simulink model "MIMO"  (R2024a)
settings: Solver=VariableStepAuto  StartTime=0.0  StopTime=20  RelTol=1e-3
undefined symbols (not defined in the file or in its folder): BOOL, DINT, slplc
(part 1 of 5)
settings Model: PLCLadderLogicAnimation=on  Creator=Jack Vranicar  LastModifiedBy=Jack Vranicar

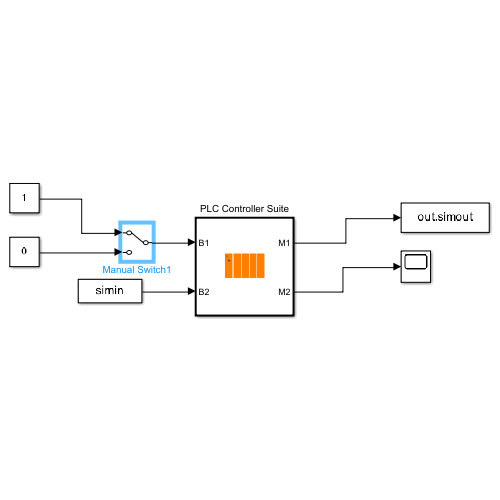
[thumbnail: Simulink's stored preview of the top-level diagram]
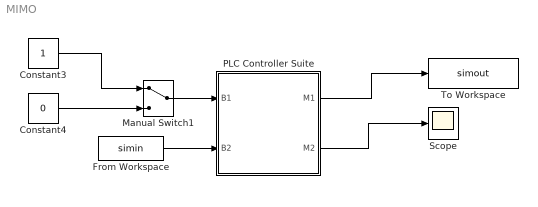
== system MIMO ==
  Constant3 : Constant  OutDataTypeStr=boolean
  Constant4 : Constant  Value=0  OutDataTypeStr=boolean
  From Workspace : FromWorkspace  VariableName=simin
  Manual Switch1 : ManualSwitch
  PLC Controller Suite : Subsystem  TreatAsAtomicUnit=on  mask{PLCBlockType=PLCController, PLCPOUType=PLC Controller}
      mask init:
      | slplc.callbacks.initController(gcb);
      settings: OpenFcn=slplc.callbacks.openPOUBlock(gcb);
      mask Help: web([docroot '/plccoder/ref/plccontrollersuite' '.html']);
      mask DialogControl PLCBlockTitle Prompt: PLC Controller Block
  Scope : Scope
  To Workspace : ToWorkspace  VariableName=simout  SaveFormat=Timeseries  SampleTime=-1
  wires:
  PLC Controller Suite/2(M2) -> Scope/1
  PLC Controller Suite/1(M1) -> To Workspace/1
  Constant4/1 -> Manual Switch1/2
  Constant3/1 -> Manual Switch1/1
  From Workspace/1 -> PLC Controller Suite/2(B2)
  Manual Switch1/1 -> PLC Controller Suite/1(B1)

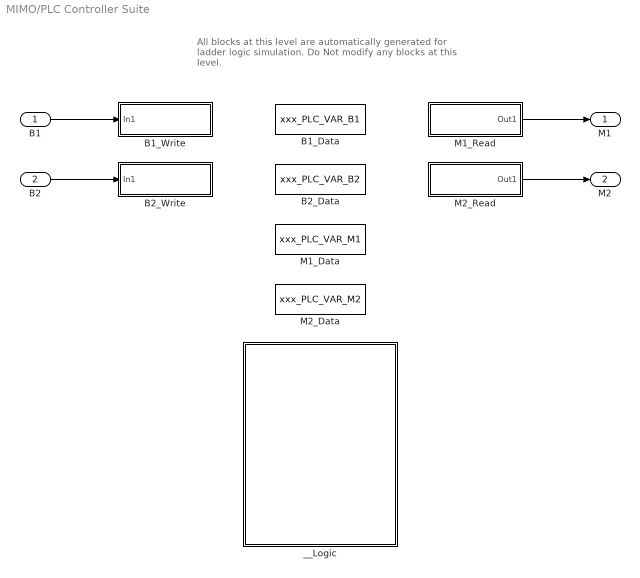
== system MIMO/PLC Controller Suite ==
  note: All blocks at this level are automatically generated for ladder logic simulation.
      | Do Not modify any blocks at this level.
  B1 : Inport  OutDataTypeStr=boolean
  B2 : Inport  Port=2  OutDataTypeStr=boolean
  B1_Data : DataStoreMemory  Tag=POUVariable  Priority=10  DataStoreName=xxx_PLC_VAR_B1  ShowAdditionalParam=off  OutDataTypeStr=boolean  Dimensions=1
  B1_Write : Subsystem  Priority=11  DisableCoverage=on  TreatAsAtomicUnit=on  mask{PLCOperandTag=B1, PLCOperandExpression=xxx_PLC_VAR_B1, PLCBlockType=VarWrite, PLCPOUType=VarWrite}
      mask prompts: PLCOperandTag "Operand Tag:"
      mask init:
      | slplc.callbacks.initInstruction(gcb);
      mask Help: web([docroot '/plccoder/ref/varwrite' '.html']);
      mask DialogControl PLCBlockTitle Prompt: Variable Write
      mask Display: disp(get_param(gcb, 'PLCOperandTag'));
  B2_Data : DataStoreMemory  Tag=POUVariable  Priority=10  DataStoreName=xxx_PLC_VAR_B2  ShowAdditionalParam=off  OutDataTypeStr=boolean  Dimensions=1
  B2_Write : Subsystem  Priority=11  DisableCoverage=on  TreatAsAtomicUnit=on  mask{PLCOperandTag=B2, PLCOperandExpression=xxx_PLC_VAR_B2, PLCBlockType=VarWrite, PLCPOUType=VarWrite}
      mask prompts: PLCOperandTag "Operand Tag:"
      mask init:
      | slplc.callbacks.initInstruction(gcb);
      mask Help: web([docroot '/plccoder/ref/varwrite' '.html']);
      mask DialogControl PLCBlockTitle Prompt: Variable Write
      mask Display: disp(get_param(gcb, 'PLCOperandTag'));
  M1_Data : DataStoreMemory  Tag=POUVariable  Priority=10  DataStoreName=xxx_PLC_VAR_M1  ShowAdditionalParam=off  OutDataTypeStr=boolean  Dimensions=1
  M1_Read : Subsystem  Priority=13  DisableCoverage=on  TreatAsAtomicUnit=on  mask{PLCOperandTag=M1, PLCOperandExpression=xxx_PLC_VAR_M1, PLCBlockType=VarRead, PLCPOUType=VarRead}
      mask prompts: PLCOperandTag "Operand Tag"
      mask init:
      | block = gcb;
      | maskObj = Simulink.Mask.get(block);
      | maskObj.Display = sprintf('disp(''%s'');', PLCOperandTag);
      | slplc.callbacks.initInstruction(gcb);
      mask Help: web([docroot '/plccoder/ref/varread' '.html']);
      mask DialogControl PLCBlockTitle Prompt: Variable Read
      mask Display: disp('M1');
  M2_Data : DataStoreMemory  Tag=POUVariable  Priority=10  DataStoreName=xxx_PLC_VAR_M2  ShowAdditionalParam=off  OutDataTypeStr=boolean  Dimensions=1
  M2_Read : Subsystem  Priority=13  DisableCoverage=on  TreatAsAtomicUnit=on  mask{PLCOperandTag=M2, PLCOperandExpression=xxx_PLC_VAR_M2, PLCBlockType=VarRead, PLCPOUType=VarRead}
      mask prompts: PLCOperandTag "Operand Tag"
      mask init:
      | block = gcb;
      | maskObj = Simulink.Mask.get(block);
      | maskObj.Display = sprintf('disp(''%s'');', PLCOperandTag);
      | slplc.callbacks.initInstruction(gcb);
      mask Help: web([docroot '/plccoder/ref/varread' '.html']);
      mask DialogControl PLCBlockTitle Prompt: Variable Read
      mask Display: disp('M2');
  __Logic : Subsystem  Priority=12  TreatAsAtomicUnit=on
  M1 : Outport
  M2 : Outport  Port=2
  wires:
  B1/1 -> B1_Write/1(In1)
  B2/1 -> B2_Write/1(In1)
  M1_Read/1(Out1) -> M1/1
  M2_Read/1(Out1) -> M2/1

== system MIMO/PLC Controller Suite/B1_Write ==
  In1 : Inport
  __CoreVarWrite : Subsystem  Tag=CoreVarWriteBlock  DisableCoverage=on  TreatAsAtomicUnit=on  mask{PLCBlockType=CoreVarWrite}
      mask init:
      | slplc.callbacks.initCoreVariable(gcb, 'write');
      mask DialogControl PLCBlockTitle Prompt: Core Variable Write
  wires:
  In1/1 -> __CoreVarWrite/1(u)

== system MIMO/PLC Controller Suite/B2_Write ==
  In1 : Inport
  __CoreVarWrite : Subsystem  Tag=CoreVarWriteBlock  DisableCoverage=on  TreatAsAtomicUnit=on  mask{PLCBlockType=CoreVarWrite}
      mask init:
      | slplc.callbacks.initCoreVariable(gcb, 'write');
      mask DialogControl PLCBlockTitle Prompt: Core Variable Write
  wires:
  In1/1 -> __CoreVarWrite/1(u)

== system MIMO/PLC Controller Suite/M1_Read ==
  __CoreVarRead : Subsystem  Tag=CoreVarReadBlock  DisableCoverage=on  TreatAsAtomicUnit=on  mask{PLCBlockType=CoreVarRead}
      mask init:
      | slplc.callbacks.initCoreVariable(gcb, 'read');
      mask DialogControl PLCBlockTitle Prompt: Core Variable Read
  Out1 : Outport  VectorParamsAs1DForOutWhenUnconnected=off
  wires:
  __CoreVarRead/1(y) -> Out1/1

== system MIMO/PLC Controller Suite/M2_Read ==
  __CoreVarRead : Subsystem  Tag=CoreVarReadBlock  DisableCoverage=on  TreatAsAtomicUnit=on  mask{PLCBlockType=CoreVarRead}
      mask init:
      | slplc.callbacks.initCoreVariable(gcb, 'read');
      mask DialogControl PLCBlockTitle Prompt: Core Variable Read
  Out1 : Outport  VectorParamsAs1DForOutWhenUnconnected=off
  wires:
  __CoreVarRead/1(y) -> Out1/1

== system MIMO/PLC Controller Suite/__Logic ==
  Controller Tags : Subsystem  Tag=ControllerVariableSS  DisableCoverage=on  TreatAsAtomicUnit=on  mask{PLCVarB1Name=B1, PLCVarB1Address=<empty>, PLCVarB1Mapping=Input Symbol, PLCVarB1PortIndex=1, PLCVarB1DataType=boolean, PLCVarB1Size=1, PLCVarB1InitialValue=0, PLCVarB1ToDelete=off, PLCVarB2Name=B2, PLCVarB2Address=<empty>, PLCVarB2Mapping=Input Symbol, PLCVarB2PortIndex=2, PLCVarB2DataType=boolean, PLCVarB2Size=1, PLCVarB2InitialValue=0, PLCVarB2ToDelete=off, PLCVarM1Name=M1, PLCVarM1Address=<empty>, PLCVarM1Mapping=Output Symbol, PLCVarM1PortIndex=1, PLCVarM1DataType=boolean, PLCVarM1Size=1, PLCVarM1InitialValue=0, PLCVarM1ToDelete=off, PLCVarM2Name=M2, PLCVarM2Address=<empty>, PLCVarM2Mapping=Output Symbol, PLCVarM2PortIndex=2, PLCVarM2DataType=boolean, PLCVarM2Size=1, PLCVarM2InitialValue=0, PLCVarM2ToDelete=off}
      mask init:
      | slplc.callbacks.initControllerVarSS(gcb);
      settings: OpenFcn=slplc.callbacks.openControllerVariableSS(gcb);
      mask Help: web([docroot '/plccoder/ref/controllertags' '.html']);
      mask TypeOptions PLCVarB1Mapping: Global Variable | Input Symbol | Output Symbol
      mask Callback PLCVarB1Mapping: slplc.callbacks.updateControllerVarSS(gcb);
      mask TypeOptions PLCVarB1PortIndex: 1 | 2 | 3 | 4
      mask TypeOptions PLCVarB2Mapping: Global Variable | Input Symbol | Output Symbol
      mask Callback PLCVarB2Mapping: slplc.callbacks.updateControllerVarSS(gcb);
      mask TypeOptions PLCVarB2PortIndex: 1 | 2 | 3 | 4
      mask TypeOptions PLCVarM1Mapping: Global Variable | Input Symbol | Output Symbol
      mask Callback PLCVarM1Mapping: slplc.callbacks.updateControllerVarSS(gcb);
      mask TypeOptions PLCVarM1PortIndex: 1 | 2 | 3 | 4
      mask TypeOptions PLCVarM2Mapping: Global Variable | Input Symbol | Output Symbol
      mask Callback PLCVarM2Mapping: slplc.callbacks.updateControllerVarSS(gcb);
      mask TypeOptions PLCVarM2PortIndex: 1 | 2 | 3 | 4
      mask DialogControl PLCBlockTitle Prompt: Global Variable and Symbol Spreadsheet
      mask DialogControl PLCVarListHeaderName Prompt: Name
      mask DialogControl PLCVarListHeaderAddress Prompt: Address (At)
      mask DialogControl PLCVarListHeaderMapping Prompt: Mapping Type
      mask DialogControl PLCVarListHeaderPortIndex Prompt: Port
      mask DialogControl PLCVarListHeaderDataType Prompt: Data Type
      mask DialogControl PLCVarListHeaderSize Prompt: Size
      mask DialogControl PLCVarListHeaderInitialValue Prompt: Initial Value
      mask DialogControl PLCVarListHeaderToDelete Prompt: Delete
  Task : Subsystem  TreatAsAtomicUnit=on  mask{PLCBlockType=Task, PLCPOUType=Task, PLCTaskWatchDog=0}
      settings: OpenFcn=slplc.callbacks.openTaskBlock(gcb);
      mask Help: web([docroot '/plccoder/ref/task' '.html']);
      mask DialogControl PLCBlockTitle Prompt: Task
  Up to Parent POU : Subsystem  DisableCoverage=on  TreatAsAtomicUnit=on  mask{PLCBlockType=OpenParentPOU}
      settings: OpenFcn=slplc.callbacks.openParentPOUBlock(gcb);
      mask Help: web([docroot '/plccoder/ref/uptoparentpou' '.html']);
      mask DialogControl PLCBlockTitle Prompt: Add Single Rung

== system MIMO/PLC Controller Suite/B1_Write/__CoreVarWrite ==
  u : Inport
  DataWrite : DataStoreWrite  DataStoreName=xxx_PLC_VAR_B1  IndexOptions=Index vector (dialog)  Indices=1  OutputSizes=1
  wires:
  u/1 -> DataWrite/1

== system MIMO/PLC Controller Suite/B2_Write/__CoreVarWrite ==
  u : Inport
  DataWrite : DataStoreWrite  DataStoreName=xxx_PLC_VAR_B2  IndexOptions=Index vector (dialog)  Indices=1  OutputSizes=1
  wires:
  u/1 -> DataWrite/1

== system MIMO/PLC Controller Suite/M1_Read/__CoreVarRead ==
  DataRead : DataStoreRead  DataStoreName=xxx_PLC_VAR_M1  IndexOptions=Index vector (dialog)  Indices=1  OutputSizes=1
  y : Outport  VectorParamsAs1DForOutWhenUnconnected=off
  wires:
  DataRead/1 -> y/1

== system MIMO/PLC Controller Suite/M2_Read/__CoreVarRead ==
  DataRead : DataStoreRead  DataStoreName=xxx_PLC_VAR_M2  IndexOptions=Index vector (dialog)  Indices=1  OutputSizes=1
  y : Outport  VectorParamsAs1DForOutWhenUnconnected=off
  wires:
  DataRead/1 -> y/1

== system MIMO/PLC Controller Suite/__Logic/Controller Tags ==

== system MIMO/PLC Controller Suite/__Logic/Task ==
  Program : Subsystem  TreatAsAtomicUnit=on  mask{PLCPOUType=Program, PLCPOULanguage=LD, PLCBlockType=LDProgram}
      mask prompts: PLCPOUType "POU Type:"
      mask init:
      | slplc.callbacks.initProgram(gcb);
      settings: OpenFcn=slplc.callbacks.openPOUBlock(gcb);
      mask Help: web([docroot '/plccoder/ref/ldprogram' '.html']);
      mask DialogControl PLCBlockTitle Prompt: Program
      mask DialogControl PLCEditPOU Prompt: Edit POU
      mask DialogControl PLCEditInterface Prompt: Edit Variables
  Up to Parent POU : Subsystem  DisableCoverage=on  TreatAsAtomicUnit=on  mask{PLCBlockType=OpenParentPOU}
      settings: OpenFcn=slplc.callbacks.openParentPOUBlock(gcb);
      mask Help: web([docroot '/plccoder/ref/uptoparentpou' '.html']);
      mask DialogControl PLCBlockTitle Prompt: Add Single Rung

== system MIMO/PLC Controller Suite/__Logic/Up to Parent POU ==

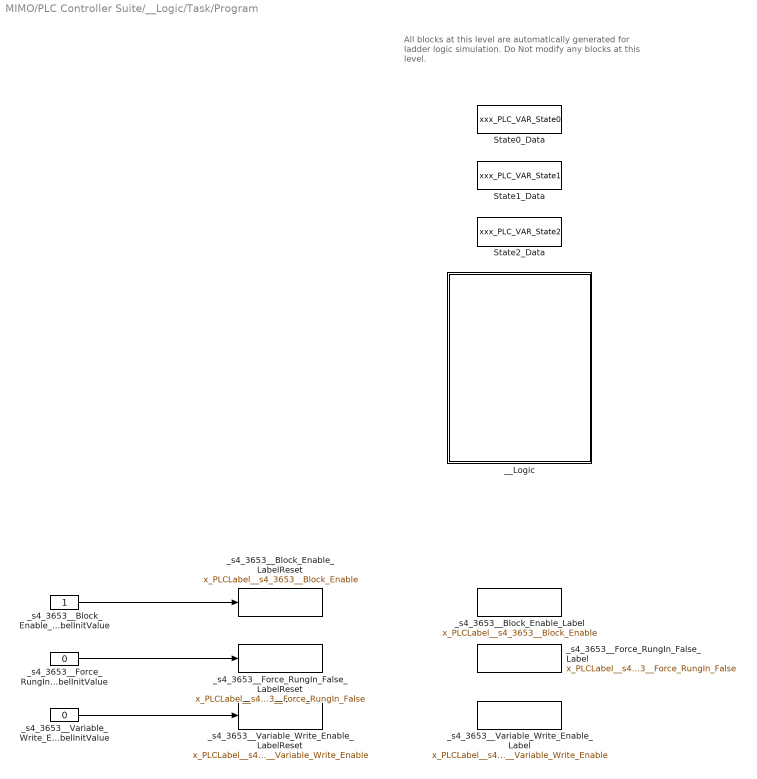
== system MIMO/PLC Controller Suite/__Logic/Task/Program ==
  note: All blocks at this level are automatically generated for ladder logic simulation.
      | Do Not modify any blocks at this level.
  State0_Data : DataStoreMemory  Tag=POUVariable  Priority=10  DataStoreName=xxx_PLC_VAR_State0  InitialValue=1  ShowAdditionalParam=off  OutDataTypeStr=BOOL  Dimensions=1
  State1_Data : DataStoreMemory  Tag=POUVariable  Priority=10  DataStoreName=xxx_PLC_VAR_State1  InitialValue=false  ShowAdditionalParam=off  OutDataTypeStr=BOOL  Dimensions=1
  State2_Data : DataStoreMemory  Tag=POUVariable  Priority=10  DataStoreName=xxx_PLC_VAR_State2  InitialValue=false  ShowAdditionalParam=off  OutDataTypeStr=BOOL  Dimensions=1
  __Logic : Subsystem  Priority=12  TreatAsAtomicUnit=on
  _s4_3653__Block_Enable_Label : DataStoreMemory  Priority=10  DataStoreName=x_PLCLabel__s4_3653__Block_Enable  InitialValue=1  ShowAdditionalParam=off  OutDataTypeStr=BOOL  Dimensions=1
  _s4_3653__Block_Enable_LabelInitValue : Constant  OutDataTypeStr=BOOL
  _s4_3653__Block_Enable_LabelReset : DataStoreWrite  Priority=11  DataStoreName=x_PLCLabel__s4_3653__Block_Enable  IndexOptions=Index vector (dialog)  Indices=1  OutputSizes=1
  _s4_3653__Force_RungIn_False_Label : DataStoreMemory  Priority=10  DataStoreName=x_PLCLabel__s4_3653__Force_RungIn_False  ShowAdditionalParam=off  OutDataTypeStr=BOOL  Dimensions=1
  _s4_3653__Force_RungIn_False_LabelInitValue : Constant  Value=0  OutDataTypeStr=BOOL
  _s4_3653__Force_RungIn_False_LabelReset : DataStoreWrite  Priority=11  DataStoreName=x_PLCLabel__s4_3653__Force_RungIn_False  IndexOptions=Index vector (dialog)  Indices=1  OutputSizes=1
  _s4_3653__Variable_Write_Enable_Label : DataStoreMemory  Priority=10  DataStoreName=x_PLCLabel__s4_3653__Variable_Write_Enable  ShowAdditionalParam=off  OutDataTypeStr=BOOL  Dimensions=1
  _s4_3653__Variable_Write_Enable_LabelInitValue : Constant  Value=0  OutDataTypeStr=BOOL
  _s4_3653__Variable_Write_Enable_LabelReset : DataStoreWrite  Priority=11  DataStoreName=x_PLCLabel__s4_3653__Variable_Write_Enable  IndexOptions=Index vector (dialog)  Indices=1  OutputSizes=1
  wires:
  _s4_3653__Block_Enable_LabelInitValue/1 -> _s4_3653__Block_Enable_LabelReset/1
  _s4_3653__Variable_Write_Enable_LabelInitValue/1 -> _s4_3653__Variable_Write_Enable_LabelReset/1
  _s4_3653__Force_RungIn_False_LabelInitValue/1 -> _s4_3653__Force_RungIn_False_LabelReset/1

== system MIMO/PLC Controller Suite/__Logic/Task/Up to Parent POU ==

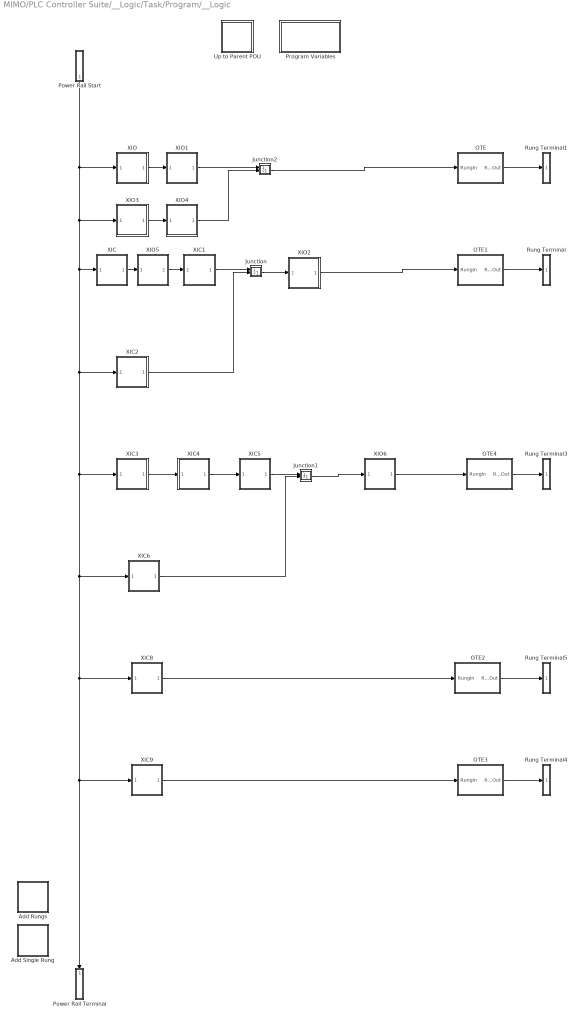
== system MIMO/PLC Controller Suite/__Logic/Task/Program/__Logic ==
  Add Rungs : Subsystem  DisableCoverage=on  TreatAsAtomicUnit=on  mask{PLCRungNumberToAdd=2, PLCBlockType=AddRungs}
      mask prompts: PLCRungNumberToAdd "Rung Number:"
      mask Help: web([docroot '/plccoder/ref/addrungs' '.html']);
      mask DialogControl PLCAddRungs Prompt: Add Rungs
      mask DialogControl PLCRungAddButton Prompt: Add
      mask DialogControl PLCRungAddButton Callback: slplc.callbacks.addLadderRungs(gcb);
      mask Display: disp(sprintf(['Add' newline 'Rungs']));
  Add Single Rung : Subsystem  DisableCoverage=on  TreatAsAtomicUnit=on  mask{PLCRungNumberToAdd=1, PLCBlockType=AddSingleRung}
      settings: OpenFcn=slplc.callbacks.addLadderRungs(gcb);
      mask Help: web([docroot '/plccoder/ref/addsinglerung' '.html']);
      mask DialogControl PLCAddRung Prompt: Add Single Rung
      mask Display: disp(sprintf(['Add' newline '1 Rung']));
  Junction : Subsystem  Priority=13  DisableCoverage=on  TreatAsAtomicUnit=on  mask{PLCBlockType=Junction, PLCPOUType=BranchJunction}
      mask Help: web([docroot '/plccoder/ref/junction' '.html']);
      mask DialogControl PLCBlockTitle Prompt: Rung Merge Point
      mask DialogControl PLCBlockDesc Prompt: This is the ladder diagram rung merge point.
  Junction1 : Subsystem  Priority=21  DisableCoverage=on  TreatAsAtomicUnit=on  mask{PLCBlockType=Junction, PLCPOUType=BranchJunction}
      mask Help: web([docroot '/plccoder/ref/junction' '.html']);
      mask DialogControl PLCBlockTitle Prompt: Rung Merge Point
      mask DialogControl PLCBlockDesc Prompt: This is the ladder diagram rung merge point.
  Junction2 : Subsystem  Priority=6  DisableCoverage=on  TreatAsAtomicUnit=on  mask{PLCBlockType=Junction, PLCPOUType=BranchJunction}
      mask Help: web([docroot '/plccoder/ref/junction' '.html']);
      mask DialogControl PLCBlockTitle Prompt: Rung Merge Point
      mask DialogControl PLCBlockDesc Prompt: This is the ladder diagram rung merge point.
  OTE : Subsystem  Priority=7  TreatAsAtomicUnit=on  mask{PLCOperandTag=State0, PLCBlockType=OTE, PLCPOUType=Coil, PLCOperandExpression=xxx_PLC_VAR_State0}
      mask prompts: PLCOperandTag "Operand Tag:"
      mask init:
      | slplc.callbacks.initInstruction(gcb);
      settings: AttributesFormatString=%<PLCOperandTag>
      mask Help: web([docroot '/plccoder/ref/ote' '.html']);
      mask DialogControl PLCBlockTitle Prompt: Output Energize (OTE)
  OTE1 : Subsystem  Priority=15  TreatAsAtomicUnit=on  mask{PLCOperandTag=State1, PLCBlockType=OTE, PLCPOUType=Coil, PLCOperandExpression=xxx_PLC_VAR_State1}
      mask prompts: PLCOperandTag "Operand Tag:"
      mask init:
      | slplc.callbacks.initInstruction(gcb);
      settings: AttributesFormatString=%<PLCOperandTag>
      mask Help: web([docroot '/plccoder/ref/ote' '.html']);
      mask DialogControl PLCBlockTitle Prompt: Output Energize (OTE)
  OTE2 : Subsystem  Priority=26  TreatAsAtomicUnit=on  mask{PLCOperandTag=M1, PLCBlockType=OTE, PLCPOUType=Coil, PLCOperandExpression=xxx_PLC_VAR_M1}
      mask prompts: PLCOperandTag "Operand Tag:"
      mask init:
      | slplc.callbacks.initInstruction(gcb);
      settings: AttributesFormatString=%<PLCOperandTag>
      mask Help: web([docroot '/plccoder/ref/ote' '.html']);
      mask DialogControl PLCBlockTitle Prompt: Output Energize (OTE)
  OTE3 : Subsystem  Priority=29  TreatAsAtomicUnit=on  mask{PLCOperandTag=M2, PLCBlockType=OTE, PLCPOUType=Coil, PLCOperandExpression=xxx_PLC_VAR_M2}
      mask prompts: PLCOperandTag "Operand Tag:"
      mask init:
      | slplc.callbacks.initInstruction(gcb);
      settings: AttributesFormatString=%<PLCOperandTag>
      mask Help: web([docroot '/plccoder/ref/ote' '.html']);
      mask DialogControl PLCBlockTitle Prompt: Output Energize (OTE)
  OTE4 : Subsystem  Priority=23  TreatAsAtomicUnit=on  mask{PLCOperandTag=State2, PLCBlockType=OTE, PLCPOUType=Coil, PLCOperandExpression=xxx_PLC_VAR_State2}
      mask prompts: PLCOperandTag "Operand Tag:"
      mask init:
      | slplc.callbacks.initInstruction(gcb);
      settings: AttributesFormatString=%<PLCOperandTag>
      mask Help: web([docroot '/plccoder/ref/ote' '.html']);
      mask DialogControl PLCBlockTitle Prompt: Output Energize (OTE)
  Power Rail Start : Subsystem  Priority=1  DisableCoverage=on  TreatAsAtomicUnit=on  mask{PLCBlockType=PowerRailStart}
      mask Help: web([docroot '/plccoder/ref/powerrailstart' '.html']);
      mask DialogControl PLCBlockTitle Prompt: Power Rail Start
      mask DialogControl PLCBlockDesc Prompt: This is the ladder diagram left power rail start block.
  Power Rail Terminal : Subsystem  DisableCoverage=on  TreatAsAtomicUnit=on  mask{PLCBlockType=PowerRailTerminal}
      mask Help: web([docroot '/plccoder/ref/powerrailterminal' '.html']);
      mask DialogControl PLCBlockTitle Prompt: Power Rail Terminal
      mask DialogControl PLCBlockDesc Prompt: This is the ladder diagram left power rail terminal block.
  Program Variables : Subsystem  Tag=ProgramVariableSS  DisableCoverage=on  TreatAsAtomicUnit=on  mask{PLCVarState0Name=State0, PLCVarState0Scope=Local, PLCVarState0PortType=Hidden, PLCVarState0PortIndex=7, PLCVarState0DataType=BOOL, PLCVarState0Size=1, PLCVarState0InitialValue=1, PLCVarState0ToDelete=off, PLCVarState1Name=State1, PLCVarState1Scope=Local, PLCVarState1PortType=Hidden, PLCVarState1PortIndex=7, PLCVarState1DataType=BOOL, PLCVarState1Size=1, PLCVarState1InitialValue=false, PLCVarState1ToDelete=off, PLCVarState2Name=State2, PLCVarState2Scope=Local, PLCVarState2PortType=Hidden, PLCVarState2PortIndex=7, PLCVarState2DataType=BOOL, PLCVarState2Size=1, PLCVarState2InitialValue=false, PLCVarState2ToDelete=off, PLCVarB1Name=B1, PLCVarB1Scope=External, PLCVarB1PortType=Hidden, PLCVarB1PortIndex=7, PLCVarB1DataType=DINT, PLCVarB1Size=-1, PLCVarB1InitialValue=0, PLCVarB1ToDelete=off, PLCVarB2Name=B2, PLCVarB2Scope=External, PLCVarB2PortType=Hidden, PLCVarB2PortIndex=7, PLCVarB2DataType=DINT, PLCVarB2Size=-1, PLCVarB2InitialValue=0, PLCVarB2ToDelete=off, PLCVarM1Name=M1, PLCVarM1Scope=External, PLCVarM1PortType=Hidden, PLCVarM1PortIndex=7, PLCVarM1DataType=DINT, PLCVarM1Size=-1, PLCVarM1InitialValue=0, PLCVarM1ToDelete=off, PLCVarM2Name=M2, PLCVarM2Scope=External, PLCVarM2PortType=Hidden, PLCVarM2PortIndex=7, PLCVarM2DataType=DINT, PLCVarM2Size=-1, PLCVarM2InitialValue=0, PLCVarM2ToDelete=off}
      mask init:
      | slplc.callbacks.initPOUVarSS(gcb);
      settings: OpenFcn=slplc.callbacks.openProgramVariableSS(gcb);
      mask Help: web([docroot '/plccoder/ref/programvariables' '.html']);
      mask TypeOptions PLCVarState0Scope: Local | External
      mask Callback PLCVarState0Scope: slplc.callbacks.updatePOUVarSS(gcb);
      mask TypeOptions PLCVarState0PortType: Hidden | Inport | Outport
      mask Callback PLCVarState0PortType: slplc.callbacks.updatePOUVarSS(gcb);
      mask TypeOptions PLCVarState0PortIndex: 1 | 2 | 3 | 4 | 5 | 6 | 7
      mask TypeOptions PLCVarState1Scope: Local | External
      mask Callback PLCVarState1Scope: slplc.callbacks.updatePOUVarSS(gcb);
      mask TypeOptions PLCVarState1PortType: Hidden | Inport | Outport
      mask Callback PLCVarState1PortType: slplc.callbacks.updatePOUVarSS(gcb);
      mask TypeOptions PLCVarState1PortIndex: 1 | 2 | 3 | 4 | 5 | 6 | 7
      mask TypeOptions PLCVarState2Scope: Local | External
      mask Callback PLCVarState2Scope: slplc.callbacks.updatePOUVarSS(gcb);
      mask TypeOptions PLCVarState2PortType: Hidden | Inport | Outport
      mask Callback PLCVarState2PortType: slplc.callbacks.updatePOUVarSS(gcb);
      mask TypeOptions PLCVarState2PortIndex: 1 | 2 | 3 | 4 | 5 | 6 | 7
      mask TypeOptions PLCVarB1Scope: Local | External
      mask Callback PLCVarB1Scope: slplc.callbacks.updatePOUVarSS(gcb);
      mask TypeOptions PLCVarB1PortType: Hidden | Inport | Outport
      mask Callback PLCVarB1PortType: slplc.callbacks.updatePOUVarSS(gcb);
      mask TypeOptions PLCVarB1PortIndex: 1 | 2 | 3 | 4 | 5 | 6 | 7
      mask TypeOptions PLCVarB2Scope: Local | External
      mask Callback PLCVarB2Scope: slplc.callbacks.updatePOUVarSS(gcb);
      mask TypeOptions PLCVarB2PortType: Hidden | Inport | Outport
      mask Callback PLCVarB2PortType: slplc.callbacks.updatePOUVarSS(gcb);
      mask TypeOptions PLCVarB2PortIndex: 1 | 2 | 3 | 4 | 5 | 6 | 7
      mask TypeOptions PLCVarM1Scope: Local | External
      mask Callback PLCVarM1Scope: slplc.callbacks.updatePOUVarSS(gcb);
      mask TypeOptions PLCVarM1PortType: Hidden | Inport | Outport
      mask Callback PLCVarM1PortType: slplc.callbacks.updatePOUVarSS(gcb);
      mask TypeOptions PLCVarM1PortIndex: 1 | 2 | 3 | 4 | 5 | 6 | 7
      mask TypeOptions PLCVarM2Scope: Local | External
      mask Callback PLCVarM2Scope: slplc.callbacks.updatePOUVarSS(gcb);
      mask TypeOptions PLCVarM2PortType: Hidden | Inport | Outport
      mask Callback PLCVarM2PortType: slplc.callbacks.updatePOUVarSS(gcb);
      mask TypeOptions PLCVarM2PortIndex: 1 | 2 | 3 | 4 | 5 | 6 | 7
      mask DialogControl PLCBlockTitle Prompt: Program Variable Spreadsheet
      mask DialogControl PLCVarListHeaderName Prompt: Name
      mask DialogControl PLCVarListHeaderScope Prompt: Scope
      mask DialogControl PLCVarListHeaderDataType Prompt: Data Type
      mask DialogControl PLCVarListHeaderSize Prompt: Size
      mask DialogControl PLCVarListHeaderInitialValue Prompt: Initial Value
      mask DialogControl PLCVarListHeaderToDelete Prompt: Delete
  Rung Terminal : Subsystem  Priority=16  DisableCoverage=on  TreatAsAtomicUnit=on  mask{PLCRungTerminalIndex=2, PLCBlockType=RungTerminal}
      settings: AttributesFormatString=Rung %<PLCRungTerminalIndex>
      mask Help: web([docroot '/plccoder/ref/rungterminal' '.html']);
      mask DialogControl PLCBlockTitle Prompt: Rung Terminal
      mask DialogControl PLCBlockDescText Prompt: This is the ladder diagram rung terminal.
  Rung Terminal1 : Subsystem  Priority=8  DisableCoverage=on  TreatAsAtomicUnit=on  mask{PLCRungTerminalIndex=1, PLCBlockType=RungTerminal}
      settings: AttributesFormatString=Rung %<PLCRungTerminalIndex>
      mask Help: web([docroot '/plccoder/ref/rungterminal' '.html']);
      mask DialogControl PLCBlockTitle Prompt: Rung Terminal
      mask DialogControl PLCBlockDescText Prompt: This is the ladder diagram rung terminal.
  Rung Terminal3 : Subsystem  Priority=24  DisableCoverage=on  TreatAsAtomicUnit=on  mask{PLCRungTerminalIndex=3, PLCBlockType=RungTerminal}
      settings: AttributesFormatString=Rung %<PLCRungTerminalIndex>
      mask Help: web([docroot '/plccoder/ref/rungterminal' '.html']);
      mask DialogControl PLCBlockTitle Prompt: Rung Terminal
      mask DialogControl PLCBlockDescText Prompt: This is the ladder diagram rung terminal.
  Rung Terminal4 : Subsystem  Priority=30  DisableCoverage=on  TreatAsAtomicUnit=on  mask{PLCRungTerminalIndex=5, PLCBlockType=RungTerminal}
      settings: AttributesFormatString=Rung %<PLCRungTerminalIndex>
      mask Help: web([docroot '/plccoder/ref/rungterminal' '.html']);
      mask DialogControl PLCBlockTitle Prompt: Rung Terminal
      mask DialogControl PLCBlockDescText Prompt: This is the ladder diagram rung terminal.
  Rung Terminal5 : Subsystem  Priority=27  DisableCoverage=on  TreatAsAtomicUnit=on  mask{PLCRungTerminalIndex=4, PLCBlockType=RungTerminal}
      settings: AttributesFormatString=Rung %<PLCRungTerminalIndex>
      mask Help: web([docroot '/plccoder/ref/rungterminal' '.html']);
      mask DialogControl PLCBlockTitle Prompt: Rung Terminal
      mask DialogControl PLCBlockDescText Prompt: This is the ladder diagram rung terminal.
  Up to Parent POU : Subsystem  DisableCoverage=on  TreatAsAtomicUnit=on  mask{PLCBlockType=OpenParentPOU}
      settings: OpenFcn=slplc.callbacks.openParentPOUBlock(gcb);
      mask Help: web([docroot '/plccoder/ref/uptoparentpou' '.html']);
      mask DialogControl PLCBlockTitle Prompt: Add Single Rung
  XIC : Subsystem  Priority=9  TreatAsAtomicUnit=on  mask{PLCOperandTag=State0, PLCBlockType=XIC, PLCPOUType=Contact, PLCOperandExpression=xxx_PLC_VAR_State0}
      mask prompts: PLCOperandTag "Operand Tag:"
      mask init:
      | slplc.callbacks.initInstruction(gcb);
      settings: AttributesFormatString=%<PLCOperandTag>
      mask Help: web([docroot '/plccoder/ref/xic' '.html']);
      mask DialogControl PLCBlockTitle Prompt: Examine If Closed (XIC)
  XIC1 : Subsystem  Priority=11  TreatAsAtomicUnit=on  mask{PLCOperandTag=B1, PLCBlockType=XIC, PLCPOUType=Contact, PLCOperandExpression=xxx_PLC_VAR_B1}
      mask prompts: PLCOperandTag "Operand Tag:"
      mask init:
      | slplc.callbacks.initInstruction(gcb);
      settings: AttributesFormatString=%<PLCOperandTag>
      mask Help: web([docroot '/plccoder/ref/xic' '.html']);
      mask DialogControl PLCBlockTitle Prompt: Examine If Closed (XIC)
  XIC2 : Subsystem  Priority=12  TreatAsAtomicUnit=on  mask{PLCOperandTag=State1, PLCBlockType=XIC, PLCPOUType=Contact, PLCOperandExpression=xxx_PLC_VAR_State1}
      mask prompts: PLCOperandTag "Operand Tag:"
      mask init:
      | slplc.callbacks.initInstruction(gcb);
      settings: AttributesFormatString=%<PLCOperandTag>
      mask Help: web([docroot '/plccoder/ref/xic' '.html']);
      mask DialogControl PLCBlockTitle Prompt: Examine If Closed (XIC)
  XIC3 : Subsystem  Priority=17  TreatAsAtomicUnit=on  mask{PLCOperandTag=State1, PLCBlockType=XIC, PLCPOUType=Contact, PLCOperandExpression=xxx_PLC_VAR_State1}
      mask prompts: PLCOperandTag "Operand Tag:"
      mask init:
      | slplc.callbacks.initInstruction(gcb);
      settings: AttributesFormatString=%<PLCOperandTag>
      mask Help: web([docroot '/plccoder/ref/xic' '.html']);
      mask DialogControl PLCBlockTitle Prompt: Examine If Closed (XIC)
  XIC4 : Subsystem  Priority=18  TreatAsAtomicUnit=on  mask{PLCOperandTag=B1, PLCBlockType=XIC, PLCPOUType=Contact, PLCOperandExpression=xxx_PLC_VAR_B1}
      mask prompts: PLCOperandTag "Operand Tag:"
      mask init:
      | slplc.callbacks.initInstruction(gcb);
      settings: AttributesFormatString=%<PLCOperandTag>
      mask Help: web([docroot '/plccoder/ref/xic' '.html']);
      mask DialogControl PLCBlockTitle Prompt: Examine If Closed (XIC)
  XIC5 : Subsystem  Priority=19  TreatAsAtomicUnit=on  mask{PLCOperandTag=B2, PLCBlockType=XIC, PLCPOUType=Contact, PLCOperandExpression=xxx_PLC_VAR_B2}
      mask prompts: PLCOperandTag "Operand Tag:"
      mask init:
      | slplc.callbacks.initInstruction(gcb);
      settings: AttributesFormatString=%<PLCOperandTag>
      mask Help: web([docroot '/plccoder/ref/xic' '.html']);
      mask DialogControl PLCBlockTitle Prompt: Examine If Closed (XIC)
  XIC6 : Subsystem  Priority=20  TreatAsAtomicUnit=on  mask{PLCOperandTag=State2, PLCBlockType=XIC, PLCPOUType=Contact, PLCOperandExpression=xxx_PLC_VAR_State2}
      mask prompts: PLCOperandTag "Operand Tag:"
      mask init:
      | slplc.callbacks.initInstruction(gcb);
      settings: AttributesFormatString=%<PLCOperandTag>
      mask Help: web([docroot '/plccoder/ref/xic' '.html']);
      mask DialogControl PLCBlockTitle Prompt: Examine If Closed (XIC)
  XIC8 : Subsystem  Priority=25  TreatAsAtomicUnit=on  mask{PLCOperandTag=State1, PLCBlockType=XIC, PLCPOUType=Contact, PLCOperandExpression=xxx_PLC_VAR_State1}
      mask prompts: PLCOperandTag "Operand Tag:"
      mask init:
      | slplc.callbacks.initInstruction(gcb);
      settings: AttributesFormatString=%<PLCOperandTag>
      mask Help: web([docroot '/plccoder/ref/xic' '.html']);
      mask DialogControl PLCBlockTitle Prompt: Examine If Closed (XIC)
  XIC9 : Subsystem  Priority=28  TreatAsAtomicUnit=on  mask{PLCOperandTag=State2, PLCBlockType=XIC, PLCPOUType=Contact, PLCOperandExpression=xxx_PLC_VAR_State2}
      mask prompts: PLCOperandTag "Operand Tag:"
      mask init:
      | slplc.callbacks.initInstruction(gcb);
      settings: AttributesFormatString=%<PLCOperandTag>
      mask Help: web([docroot '/plccoder/ref/xic' '.html']);
      mask DialogControl PLCBlockTitle Prompt: Examine If Closed (XIC)
  XIO : Subsystem  Priority=2  TreatAsAtomicUnit=on  mask{PLCOperandExpression=xxx_PLC_VAR_State1, PLCOperandTag=State1, PLCBlockType=XIO, PLCPOUType=Contact}
      mask prompts: PLCOperandTag "Operand Tag:"
      mask init:
      | slplc.callbacks.initInstruction(gcb);
      settings: AttributesFormatString=%<PLCOperandTag>
      mask Help: web([docroot '/plccoder/ref/xio' '.html']);
      mask DialogControl PLCBlockTitle Prompt: Examine If Open (XIO)
  XIO1 : Subsystem  Priority=3  TreatAsAtomicUnit=on  mask{PLCOperandExpression=xxx_PLC_VAR_State2, PLCOperandTag=State2, PLCBlockType=XIO, PLCPOUType=Contact}
      mask prompts: PLCOperandTag "Operand Tag:"
      mask init:
      | slplc.callbacks.initInstruction(gcb);
      settings: AttributesFormatString=%<PLCOperandTag>
      mask Help: web([docroot '/plccoder/ref/xio' '.html']);
      mask DialogControl PLCBlockTitle Prompt: Examine If Open (XIO)
  XIO2 : Subsystem  Priority=14  TreatAsAtomicUnit=on  mask{PLCOperandExpression=xxx_PLC_VAR_State2, PLCOperandTag=State2, PLCBlockType=XIO, PLCPOUType=Contact}
      mask prompts: PLCOperandTag "Operand Tag:"
      mask init:
      | slplc.callbacks.initInstruction(gcb);
      settings: AttributesFormatString=%<PLCOperandTag>
      mask Help: web([docroot '/plccoder/ref/xio' '.html']);
      mask DialogControl PLCBlockTitle Prompt: Examine If Open (XIO)
  XIO3 : Subsystem  Priority=4  TreatAsAtomicUnit=on  mask{PLCOperandExpression=xxx_PLC_VAR_B1, PLCOperandTag=B1, PLCBlockType=XIO, PLCPOUType=Contact}
      mask prompts: PLCOperandTag "Operand Tag:"
      mask init:
      | slplc.callbacks.initInstruction(gcb);
      settings: AttributesFormatString=%<PLCOperandTag>
      mask Help: web([docroot '/plccoder/ref/xio' '.html']);
      mask DialogControl PLCBlockTitle Prompt: Examine If Open (XIO)
  XIO4 : Subsystem  Priority=5  TreatAsAtomicUnit=on  mask{PLCOperandExpression=xxx_PLC_VAR_B2, PLCOperandTag=B2, PLCBlockType=XIO, PLCPOUType=Contact}
      mask prompts: PLCOperandTag "Operand Tag:"
      mask init:
      | slplc.callbacks.initInstruction(gcb);
      settings: AttributesFormatString=%<PLCOperandTag>
      mask Help: web([docroot '/plccoder/ref/xio' '.html']);
      mask DialogControl PLCBlockTitle Prompt: Examine If Open (XIO)
  XIO5 : Subsystem  Priority=10  TreatAsAtomicUnit=on  mask{PLCOperandExpression=xxx_PLC_VAR_B2, PLCOperandTag=B2, PLCBlockType=XIO, PLCPOUType=Contact}
      mask prompts: PLCOperandTag "Operand Tag:"
      mask init:
      | slplc.callbacks.initInstruction(gcb);
      settings: AttributesFormatString=%<PLCOperandTag>
      mask Help: web([docroot '/plccoder/ref/xio' '.html']);
      mask DialogControl PLCBlockTitle Prompt: Examine If Open (XIO)
  XIO6 : Subsystem  Priority=22  TreatAsAtomicUnit=on  mask{PLCOperandExpression=xxx_PLC_VAR_State0, PLCOperandTag=State0, PLCBlockType=XIO, PLCPOUType=Contact}
      mask prompts: PLCOperandTag "Operand Tag:"
      mask init:
      | slplc.callbacks.initInstruction(gcb);
      settings: AttributesFormatString=%<PLCOperandTag>
      mask Help: web([docroot '/plccoder/ref/xio' '.html']);
      mask DialogControl PLCBlockTitle Prompt: Examine If Open (XIO)
  wires:
  Power Rail Start/1(PowerOut) -> Power Rail Terminal/1(PowerIn), XIC9/1(RungIn), XIC8/1(RungIn), XIC6/1(RungIn), XIC3/1(RungIn), XIC2/1(RungIn), XIC/1(RungIn), XIO3/1(RungIn), XIO/1(RungIn)
  XIO/1(RungOut) -> XIO1/1(RungIn)
  OTE/1(RungOut) -> Rung Terminal1/1(RungIn)
  XIC/1(RungOut) -> XIO5/1(RungIn)
  XIC1/1(RungOut) -> Junction/1(RungIn1)
  XIC2/1(RungOut) -> Junction/2(RungIn2)
  Junction/1(RungOut) -> XIO2/1(RungIn)
  XIO2/1(RungOut) -> OTE1/1(RungIn)
  OTE1/1(RungOut) -> Rung Terminal/1(RungIn)
  XIC3/1(RungOut) -> XIC4/1(RungIn)
  XIC4/1(RungOut) -> XIC5/1(RungIn)
  XIC5/1(RungOut) -> Junction1/1(RungIn1)
  XIC6/1(RungOut) -> Junction1/2(RungIn2)
  Junction1/1(RungOut) -> XIO6/1(RungIn)
  XIO6/1(RungOut) -> OTE4/1(RungIn)
  XIC8/1(RungOut) -> OTE2/1(RungIn)
  OTE2/1(RungOut) -> Rung Terminal5/1(RungIn)
  XIC9/1(RungOut) -> OTE3/1(RungIn)
  OTE3/1(RungOut) -> Rung Terminal4/1(RungIn)
  XIO3/1(RungOut) -> XIO4/1(RungIn)
  XIO1/1(RungOut) -> Junction2/1(RungIn1)
  XIO4/1(RungOut) -> Junction2/2(RungIn2)
  Junction2/1(RungOut) -> OTE/1(RungIn)
  XIO5/1(RungOut) -> XIC1/1(RungIn)
  OTE4/1(RungOut) -> Rung Terminal3/1(RungIn)

== system MIMO/PLC Controller Suite/__Logic/Task/Program/__Logic/Add Rungs ==

== system MIMO/PLC Controller Suite/__Logic/Task/Program/__Logic/Add Single Rung ==

== system MIMO/PLC Controller Suite/__Logic/Task/Program/__Logic/Junction ==
  RungIn1 : Inport
  RungIn2 : Inport  Port=2
  BlockEnableRead : Subsystem  DisableCoverage=on  TreatAsAtomicUnit=on  mask{PLCLabelTag=_Block_Enable, PLCBlockType=BlockEnableRead}
      mask prompts: PLCLabelTag "Label Tag:"
      mask init:
      | block = gcb;
      | maskObj = Simulink.Mask.get(block);
      | maskObj.Display = sprintf('disp(''%s'');', PLCLabelTag);
      mask Help: web([docroot '/plccoder/ref/blockenableread' '.html']);
      mask DialogControl PLCBlockTitle Prompt: Block Enable Read
      mask Display: disp('_Block_Enable');
  __Enable : Subsystem  TreatAsAtomicUnit=on
  __Format : MATLAB Function  Tag=PLC_Format_Joint  Priority=20  DisableCoverage=on  InitFcn=slplc.utils.setBlockAppearance('reset', '', {'black', 'black'});  StopFcn=slplc.utils.setBlockAppearance('reset', '', {'black', 'black'});  TreatAsAtomicUnit=on
  RungOut : Outport  VectorParamsAs1DForOutWhenUnconnected=off
  wires:
  __Enable/1(RungOut) -> RungOut/1, __Format/2(RungOut)
  RungIn2/1 -> __Enable/2(RungIn2)
  RungIn1/1 -> __Enable/1(RungIn1)
  BlockEnableRead/1(Out1) -> __Enable/Enable, __Format/1(BlockEnable)

== system MIMO/PLC Controller Suite/__Logic/Task/Program/__Logic/Junction1 ==
  RungIn1 : Inport
  RungIn2 : Inport  Port=2
  BlockEnableRead : Subsystem  DisableCoverage=on  TreatAsAtomicUnit=on  mask{PLCLabelTag=_Block_Enable, PLCBlockType=BlockEnableRead}
      mask prompts: PLCLabelTag "Label Tag:"
      mask init:
      | block = gcb;
      | maskObj = Simulink.Mask.get(block);
      | maskObj.Display = sprintf('disp(''%s'');', PLCLabelTag);
      mask Help: web([docroot '/plccoder/ref/blockenableread' '.html']);
      mask DialogControl PLCBlockTitle Prompt: Block Enable Read
      mask Display: disp('_Block_Enable');
  __Enable : Subsystem  TreatAsAtomicUnit=on
  __Format : MATLAB Function  Tag=PLC_Format_Joint  Priority=20  DisableCoverage=on  InitFcn=slplc.utils.setBlockAppearance('reset', '', {'black', 'black'});  StopFcn=slplc.utils.setBlockAppearance('reset', '', {'black', 'black'});  TreatAsAtomicUnit=on
  RungOut : Outport  VectorParamsAs1DForOutWhenUnconnected=off
  wires:
  __Enable/1(RungOut) -> RungOut/1, __Format/2(RungOut)
  RungIn2/1 -> __Enable/2(RungIn2)
  RungIn1/1 -> __Enable/1(RungIn1)
  BlockEnableRead/1(Out1) -> __Enable/Enable, __Format/1(BlockEnable)

== system MIMO/PLC Controller Suite/__Logic/Task/Program/__Logic/Junction2 ==
  RungIn1 : Inport
  RungIn2 : Inport  Port=2
  BlockEnableRead : Subsystem  DisableCoverage=on  TreatAsAtomicUnit=on  mask{PLCLabelTag=_Block_Enable, PLCBlockType=BlockEnableRead}
      mask prompts: PLCLabelTag "Label Tag:"
      mask init:
      | block = gcb;
      | maskObj = Simulink.Mask.get(block);
      | maskObj.Display = sprintf('disp(''%s'');', PLCLabelTag);
      mask Help: web([docroot '/plccoder/ref/blockenableread' '.html']);
      mask DialogControl PLCBlockTitle Prompt: Block Enable Read
      mask Display: disp('_Block_Enable');
  __Enable : Subsystem  TreatAsAtomicUnit=on
  __Format : MATLAB Function  Tag=PLC_Format_Joint  Priority=20  DisableCoverage=on  InitFcn=slplc.utils.setBlockAppearance('reset', '', {'black', 'black'});  StopFcn=slplc.utils.setBlockAppearance('reset', '', {'black', 'black'});  TreatAsAtomicUnit=on
  RungOut : Outport  VectorParamsAs1DForOutWhenUnconnected=off
  wires:
  __Enable/1(RungOut) -> RungOut/1, __Format/2(RungOut)
  RungIn2/1 -> __Enable/2(RungIn2)
  RungIn1/1 -> __Enable/1(RungIn1)
  BlockEnableRead/1(Out1) -> __Enable/Enable, __Format/1(BlockEnable)

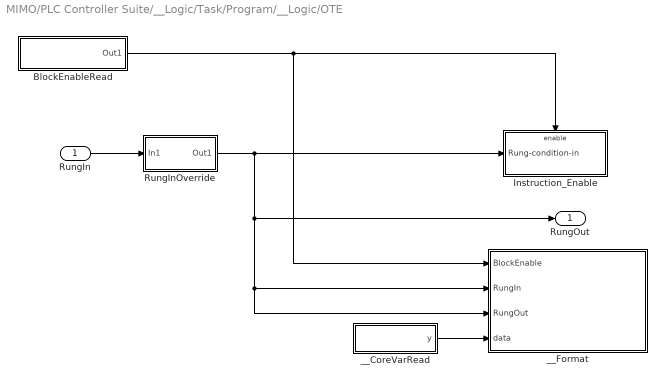
== system MIMO/PLC Controller Suite/__Logic/Task/Program/__Logic/OTE ==
  RungIn : Inport  PortDimensions=1
  BlockEnableRead : Subsystem  DisableCoverage=on  TreatAsAtomicUnit=on  mask{PLCLabelTag=_Block_Enable, PLCBlockType=BlockEnableRead}
      mask prompts: PLCLabelTag "Label Tag:"
      mask init:
      | block = gcb;
      | maskObj = Simulink.Mask.get(block);
      | maskObj.Display = sprintf('disp(''%s'');', PLCLabelTag);
      mask Help: web([docroot '/plccoder/ref/blockenableread' '.html']);
      mask DialogControl PLCBlockTitle Prompt: Block Enable Read
      mask Display: disp('_Block_Enable');
  Instruction_Enable : Subsystem  Priority=12  TreatAsAtomicUnit=on
  RungInOverride : Subsystem  DisableCoverage=on  TreatAsAtomicUnit=on
  __CoreVarRead : Subsystem  Tag=CoreVarReadBlock  DisableCoverage=on  TreatAsAtomicUnit=on  mask{PLCBlockType=CoreVarRead}
      mask init:
      | slplc.callbacks.initCoreVariable(gcb, 'read');
      mask Help: web([docroot '/plccoder/ref/__corevarread' '.html']);
      mask DialogControl PLCBlockTitle Prompt: Core Variable Read
  __Format : MATLAB Function  Tag=PLC_Format_Boolean  Priority=20  DisableCoverage=on  InitFcn=slplc.utils.setBlockAppearance('reset', '%<PLCOperandTag>');  StopFcn=slplc.utils.setBlockAppearance('reset', '%<PLCOperandTag>');  TreatAsAtomicUnit=on
  RungOut : Outport  OutDataTypeStr=BOOL  PortDimensions=1  InitialOutput=false  VectorParamsAs1DForOutWhenUnconnected=off
  wires:
  RungIn/1 -> RungInOverride/1(In1)
  BlockEnableRead/1(Out1) -> __Format/1(BlockEnable), Instruction_Enable/Enable
  RungInOverride/1(Out1) -> __Format/2(RungIn), __Format/3(RungOut), RungOut/1, Instruction_Enable/1(Rung-condition-in)
  __CoreVarRead/1(y) -> __Format/4(data)

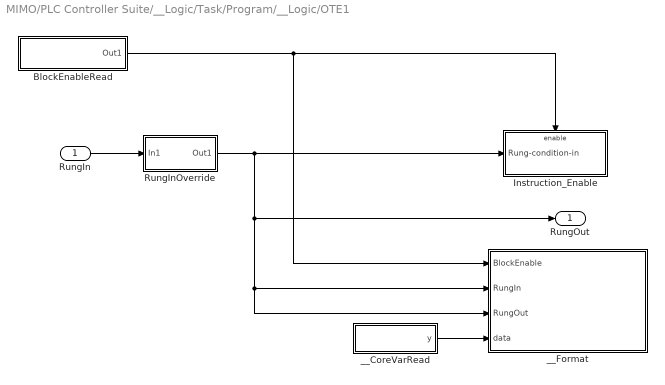
== system MIMO/PLC Controller Suite/__Logic/Task/Program/__Logic/OTE1 ==
  RungIn : Inport  PortDimensions=1
  BlockEnableRead : Subsystem  DisableCoverage=on  TreatAsAtomicUnit=on  mask{PLCLabelTag=_Block_Enable, PLCBlockType=BlockEnableRead}
      mask prompts: PLCLabelTag "Label Tag:"
      mask init:
      | block = gcb;
      | maskObj = Simulink.Mask.get(block);
      | maskObj.Display = sprintf('disp(''%s'');', PLCLabelTag);
      mask Help: web([docroot '/plccoder/ref/blockenableread' '.html']);
      mask DialogControl PLCBlockTitle Prompt: Block Enable Read
      mask Display: disp('_Block_Enable');
  Instruction_Enable : Subsystem  Priority=12  TreatAsAtomicUnit=on
  RungInOverride : Subsystem  DisableCoverage=on  TreatAsAtomicUnit=on
  __CoreVarRead : Subsystem  Tag=CoreVarReadBlock  DisableCoverage=on  TreatAsAtomicUnit=on  mask{PLCBlockType=CoreVarRead}
      mask init:
      | slplc.callbacks.initCoreVariable(gcb, 'read');
      mask Help: web([docroot '/plccoder/ref/__corevarread' '.html']);
      mask DialogControl PLCBlockTitle Prompt: Core Variable Read
  __Format : MATLAB Function  Tag=PLC_Format_Boolean  Priority=20  DisableCoverage=on  InitFcn=slplc.utils.setBlockAppearance('reset', '%<PLCOperandTag>');  StopFcn=slplc.utils.setBlockAppearance('reset', '%<PLCOperandTag>');  TreatAsAtomicUnit=on
  RungOut : Outport  OutDataTypeStr=BOOL  PortDimensions=1  InitialOutput=false  VectorParamsAs1DForOutWhenUnconnected=off
  wires:
  RungIn/1 -> RungInOverride/1(In1)
  BlockEnableRead/1(Out1) -> __Format/1(BlockEnable), Instruction_Enable/Enable
  RungInOverride/1(Out1) -> __Format/2(RungIn), __Format/3(RungOut), RungOut/1, Instruction_Enable/1(Rung-condition-in)
  __CoreVarRead/1(y) -> __Format/4(data)

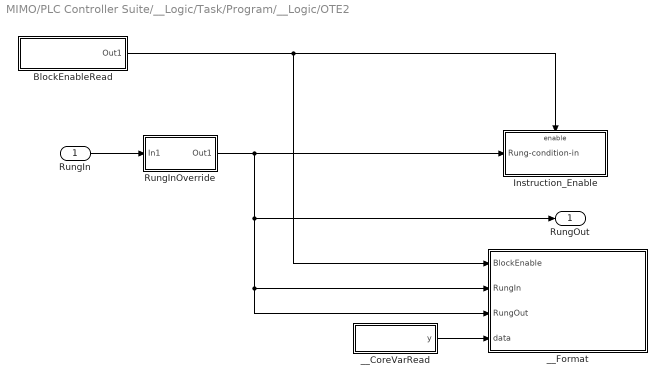
== system MIMO/PLC Controller Suite/__Logic/Task/Program/__Logic/OTE2 ==
  RungIn : Inport  PortDimensions=1
  BlockEnableRead : Subsystem  DisableCoverage=on  TreatAsAtomicUnit=on  mask{PLCLabelTag=_Block_Enable, PLCBlockType=BlockEnableRead}
      mask prompts: PLCLabelTag "Label Tag:"
      mask init:
      | block = gcb;
      | maskObj = Simulink.Mask.get(block);
      | maskObj.Display = sprintf('disp(''%s'');', PLCLabelTag);
      mask Help: web([docroot '/plccoder/ref/blockenableread' '.html']);
      mask DialogControl PLCBlockTitle Prompt: Block Enable Read
      mask Display: disp('_Block_Enable');
  Instruction_Enable : Subsystem  Priority=12  TreatAsAtomicUnit=on
  RungInOverride : Subsystem  DisableCoverage=on  TreatAsAtomicUnit=on
  __CoreVarRead : Subsystem  Tag=CoreVarReadBlock  DisableCoverage=on  TreatAsAtomicUnit=on  mask{PLCBlockType=CoreVarRead}
      mask init:
      | slplc.callbacks.initCoreVariable(gcb, 'read');
      mask Help: web([docroot '/plccoder/ref/__corevarread' '.html']);
      mask DialogControl PLCBlockTitle Prompt: Core Variable Read
  __Format : MATLAB Function  Tag=PLC_Format_Boolean  Priority=20  DisableCoverage=on  InitFcn=slplc.utils.setBlockAppearance('reset', '%<PLCOperandTag>');  StopFcn=slplc.utils.setBlockAppearance('reset', '%<PLCOperandTag>');  TreatAsAtomicUnit=on
  RungOut : Outport  OutDataTypeStr=BOOL  PortDimensions=1  InitialOutput=false  VectorParamsAs1DForOutWhenUnconnected=off
  wires:
  RungIn/1 -> RungInOverride/1(In1)
  BlockEnableRead/1(Out1) -> __Format/1(BlockEnable), Instruction_Enable/Enable
  RungInOverride/1(Out1) -> __Format/2(RungIn), __Format/3(RungOut), RungOut/1, Instruction_Enable/1(Rung-condition-in)
  __CoreVarRead/1(y) -> __Format/4(data)

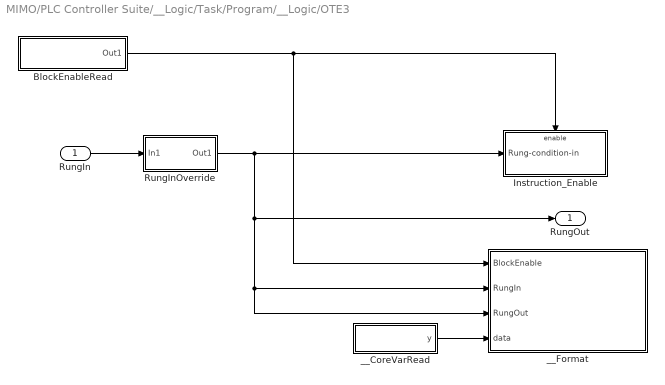
== system MIMO/PLC Controller Suite/__Logic/Task/Program/__Logic/OTE3 ==
  RungIn : Inport  PortDimensions=1
  BlockEnableRead : Subsystem  DisableCoverage=on  TreatAsAtomicUnit=on  mask{PLCLabelTag=_Block_Enable, PLCBlockType=BlockEnableRead}
      mask prompts: PLCLabelTag "Label Tag:"
      mask init:
      | block = gcb;
      | maskObj = Simulink.Mask.get(block);
      | maskObj.Display = sprintf('disp(''%s'');', PLCLabelTag);
      mask Help: web([docroot '/plccoder/ref/blockenableread' '.html']);
      mask DialogControl PLCBlockTitle Prompt: Block Enable Read
      mask Display: disp('_Block_Enable');
  Instruction_Enable : Subsystem  Priority=12  TreatAsAtomicUnit=on
  RungInOverride : Subsystem  DisableCoverage=on  TreatAsAtomicUnit=on
  __CoreVarRead : Subsystem  Tag=CoreVarReadBlock  DisableCoverage=on  TreatAsAtomicUnit=on  mask{PLCBlockType=CoreVarRead}
      mask init:
      | slplc.callbacks.initCoreVariable(gcb, 'read');
      mask Help: web([docroot '/plccoder/ref/__corevarread' '.html']);
      mask DialogControl PLCBlockTitle Prompt: Core Variable Read
  __Format : MATLAB Function  Tag=PLC_Format_Boolean  Priority=20  DisableCoverage=on  InitFcn=slplc.utils.setBlockAppearance('reset', '%<PLCOperandTag>');  StopFcn=slplc.utils.setBlockAppearance('reset', '%<PLCOperandTag>');  TreatAsAtomicUnit=on
  RungOut : Outport  OutDataTypeStr=BOOL  PortDimensions=1  InitialOutput=false  VectorParamsAs1DForOutWhenUnconnected=off
  wires:
  RungIn/1 -> RungInOverride/1(In1)
  BlockEnableRead/1(Out1) -> __Format/1(BlockEnable), Instruction_Enable/Enable
  RungInOverride/1(Out1) -> __Format/2(RungIn), __Format/3(RungOut), RungOut/1, Instruction_Enable/1(Rung-condition-in)
  __CoreVarRead/1(y) -> __Format/4(data)

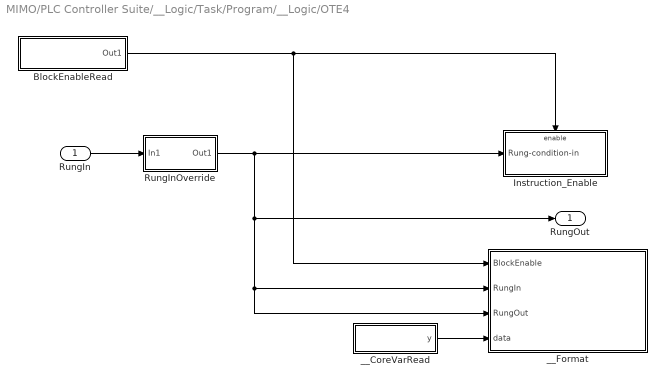
== system MIMO/PLC Controller Suite/__Logic/Task/Program/__Logic/OTE4 ==
  RungIn : Inport  PortDimensions=1
  BlockEnableRead : Subsystem  DisableCoverage=on  TreatAsAtomicUnit=on  mask{PLCLabelTag=_Block_Enable, PLCBlockType=BlockEnableRead}
      mask prompts: PLCLabelTag "Label Tag:"
      mask init:
      | block = gcb;
      | maskObj = Simulink.Mask.get(block);
      | maskObj.Display = sprintf('disp(''%s'');', PLCLabelTag);
      mask Help: web([docroot '/plccoder/ref/blockenableread' '.html']);
      mask DialogControl PLCBlockTitle Prompt: Block Enable Read
      mask Display: disp('_Block_Enable');
  Instruction_Enable : Subsystem  Priority=12  TreatAsAtomicUnit=on
  RungInOverride : Subsystem  DisableCoverage=on  TreatAsAtomicUnit=on
  __CoreVarRead : Subsystem  Tag=CoreVarReadBlock  DisableCoverage=on  TreatAsAtomicUnit=on  mask{PLCBlockType=CoreVarRead}
      mask init:
      | slplc.callbacks.initCoreVariable(gcb, 'read');
      mask Help: web([docroot '/plccoder/ref/__corevarread' '.html']);
      mask DialogControl PLCBlockTitle Prompt: Core Variable Read
  __Format : MATLAB Function  Tag=PLC_Format_Boolean  Priority=20  DisableCoverage=on  InitFcn=slplc.utils.setBlockAppearance('reset', '%<PLCOperandTag>');  StopFcn=slplc.utils.setBlockAppearance('reset', '%<PLCOperandTag>');  TreatAsAtomicUnit=on
  RungOut : Outport  OutDataTypeStr=BOOL  PortDimensions=1  InitialOutput=false  VectorParamsAs1DForOutWhenUnconnected=off
  wires:
  RungIn/1 -> RungInOverride/1(In1)
  BlockEnableRead/1(Out1) -> __Format/1(BlockEnable), Instruction_Enable/Enable
  RungInOverride/1(Out1) -> __Format/2(RungIn), __Format/3(RungOut), RungOut/1, Instruction_Enable/1(Rung-condition-in)
  __CoreVarRead/1(y) -> __Format/4(data)

== system MIMO/PLC Controller Suite/__Logic/Task/Program/__Logic/Power Rail Start ==
  PLCPowerOn : Constant  Value=true  OutDataTypeStr=BOOL
  __Format : MATLAB Function  Tag=PLC_Format_ENO  Priority=20  DisableCoverage=on  InitFcn=slplc.utils.setBlockAppearance('reset', '', {'black', 'black'});  StopFcn=slplc.utils.setBlockAppearance('reset', '', {'black', 'black'});  TreatAsAtomicUnit=on
  PowerOut : Outport  VectorParamsAs1DForOutWhenUnconnected=off
  wires:
  PLCPowerOn/1 -> __Format/1(RungOut), PowerOut/1

== system MIMO/PLC Controller Suite/__Logic/Task/Program/__Logic/Power Rail Terminal ==
  PowerIn : Inport
  Terminator3 : Terminator
  wires:
  PowerIn/1 -> Terminator3/1

== system MIMO/PLC Controller Suite/__Logic/Task/Program/__Logic/Program Variables ==

== system MIMO/PLC Controller Suite/__Logic/Task/Program/__Logic/Rung Terminal ==
  RungIn : Inport
  Terminator : Terminator
  wires:
  RungIn/1 -> Terminator/1

== system MIMO/PLC Controller Suite/__Logic/Task/Program/__Logic/Rung Terminal1 ==
  RungIn : Inport
  Terminator : Terminator
  wires:
  RungIn/1 -> Terminator/1

== system MIMO/PLC Controller Suite/__Logic/Task/Program/__Logic/Rung Terminal3 ==
  RungIn : Inport
  Terminator : Terminator
  wires:
  RungIn/1 -> Terminator/1

== system MIMO/PLC Controller Suite/__Logic/Task/Program/__Logic/Rung Terminal4 ==
  RungIn : Inport
  Terminator : Terminator
  wires:
  RungIn/1 -> Terminator/1

== system MIMO/PLC Controller Suite/__Logic/Task/Program/__Logic/Rung Terminal5 ==
  RungIn : Inport
  Terminator : Terminator
  wires:
  RungIn/1 -> Terminator/1

== system MIMO/PLC Controller Suite/__Logic/Task/Program/__Logic/Up to Parent POU ==
